simulink model "ekf_scheme_realdata"  (R2015b)
settings: Solver=ode45  StartTime=0.0  StopTime=1000  RelTol=1e-3
InitFcn:
  | script
settings Model: Creator=gianl  LastModifiedBy=gianl
settings HardwareCC: ProdWordSize=32  ProdHWDeviceType=Specified

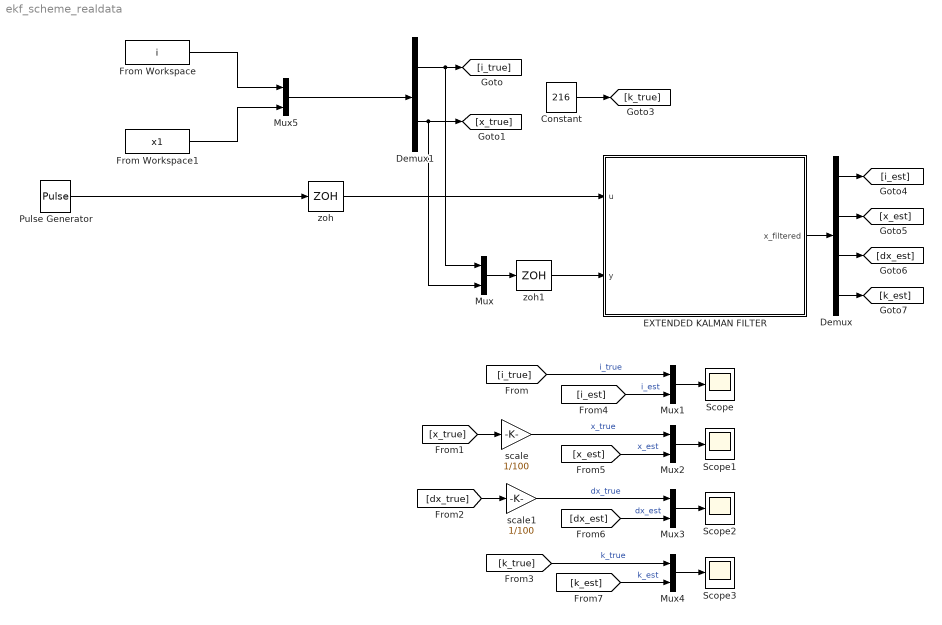
== system ekf_scheme_realdata ==
  Constant : Constant  Value=216
  Demux : Demux
  Demux1 : Demux  Outputs=2
  EXTENDED KALMAN FILTER : MATLAB Function  TreatAsAtomicUnit=on
  From Workspace : FromWorkspace  VariableName=i  SampleTime=0
  From Workspace1 : FromWorkspace  VariableName=x1  SampleTime=0
  Mux{,1..5} (6 alike) : Mux  Inputs=2
  Pulse Generator : DiscretePulseGenerator  PulseType=Time based  Amplitude=2  Period=5  PulseWidth=50  PhaseDelay=3
  Scope{,1..3} (4 alike) : Scope
  scale : Gain  Gain=1/100
  scale1 : Gain  Gain=1/100
  zoh : ZeroOrderHold  SampleTime=1/200
  zoh1 : ZeroOrderHold  SampleTime=1/200
  wires:
  zoh/1 -> EXTENDED KALMAN FILTER/1(u)
  Mux5/1 -> Demux1/1
  zoh1/1 -> EXTENDED KALMAN FILTER/2(y)
  EXTENDED KALMAN FILTER/1(x_filtered) -> Demux/1
  Mux/1 -> zoh1/1
  Demux1/1 -> Mux/1, [i_true]
  Demux1/2 -> Mux/2, [x_true]
  Constant/1 -> [k_true]
  Demux/2 -> [x_est]
  Demux/1 -> [i_est]
  Demux/3 -> [dx_est]
  Demux/4 -> [k_est]
  Mux1/1 -> Scope/1
  Mux2/1 -> Scope1/1
  Mux3/1 -> Scope2/1
  Mux4/1 -> Scope3/1
  [i_true] -> Mux1/1  "i_true"
  [x_true] -> scale/1
  [dx_true] -> scale1/1
  [k_true] -> Mux4/1  "k_true"
  [i_est] -> Mux1/2  "i_est"
  [x_est] -> Mux2/2  "x_est"
  [dx_est] -> Mux3/2  "dx_est"
  [k_est] -> Mux4/2  "k_est"
  scale/1 -> Mux2/1  "x_true"
  scale1/1 -> Mux3/1  "dx_true"
  From Workspace/1 -> Mux5/1
  From Workspace1/1 -> Mux5/2
  Pulse Generator/1 -> zoh/1

== matlab function ekf_scheme_realdata/EXTENDED KALMAN FILTER ==
  data: u input; y input; x_filtered output
function x_filtered  = ekf(u, y)
    %% Discrete Kalman filter for continous system
    % Inputs:
    % u: input to the system
    % y: output of the system
    % Output:
    % x_filtered: Kalman state estimate
    
    
    % P and xhat need to be updated each iteration
    % The other variables are parameters of the real vector.
    persistent P xhat Q R Res L M Gamma C B H
    
    if isempty(P)%First iteration, initialize values
        P = eye(4);
        xhat = [0; 0; 0; 100];
        Q = 1e-10*eye(4);
        R = diag([0.0127; 1e-10]);
        
        M = 1.8;
        C = 8.9973;
        Res = 1.3;
        L = 0.0024;
        Gamma = -2.068;
        
        B = 1/200.*[1/L; 0; 0; 0]; %Discretized Input Matrix B
        H = [1 0 0 0; 0 100 0 0]; % Output current and position
    end
    
    % Linearize the continuos system around xhat
    A = [ -Res/L,       0,              0,      0; ...
          0,            0,              1,      0; ...
        Gamma/M,        -xhat(4)/M,     -C/M,   -xhat(2)/M; ...
        0,              0,              0,      0];
    
    A = eye(4) + 1/200.*A; %Discretize A

    % Real nonlinear system computed in xhat
    f = [ -Res/L*xhat(1); ...
          xhat(3); ...
          Gamma/M*xhat(1) - xhat(4)*xhat(2)/M - C/M*xhat(3); ...
          0 ];
     
    % Discretize f 
    f = 1/200.*f;
    f = f + xhat;
    
    % Update Prediction
    x_pred = f + B*u;   % x_k+1 = f(x_k) + Bu_k
    y_pred = H*x_pred;  % y_k+1 = H*x_k+1
    
    % Update P
    P = A*P*A' + Q;
    
    % Update Kalman Gain
    K = P*H'/(H*P*H'+R);
    
    %Update Prediction
    xhat = x_pred + K*(y - y_pred);
    
    % Update P
    P = (eye(size(K*H)) - K*H)*P;
    
    % Output the state-estimate
    x_filtered = xhat;
